simulink model "Final_prob"  (R2024b)
settings: Solver=VariableStepAuto  StartTime=0.0  StopTime=12  RelTol=1e-3
undefined symbols (not defined in the file or in its folder): A, B, C, D, sigbuilder_block
settings Model: Creator=shree  LastModifiedBy=shree

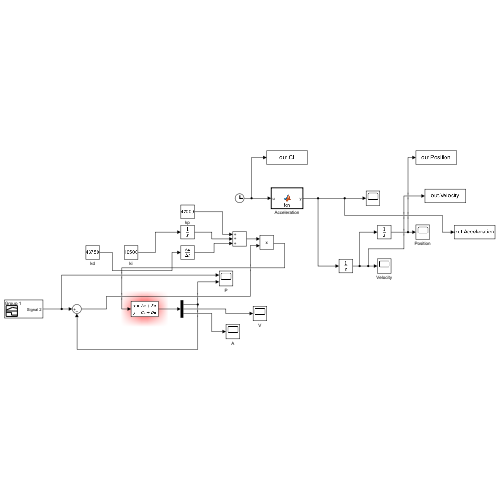
[thumbnail: Simulink's stored preview of the top-level diagram]
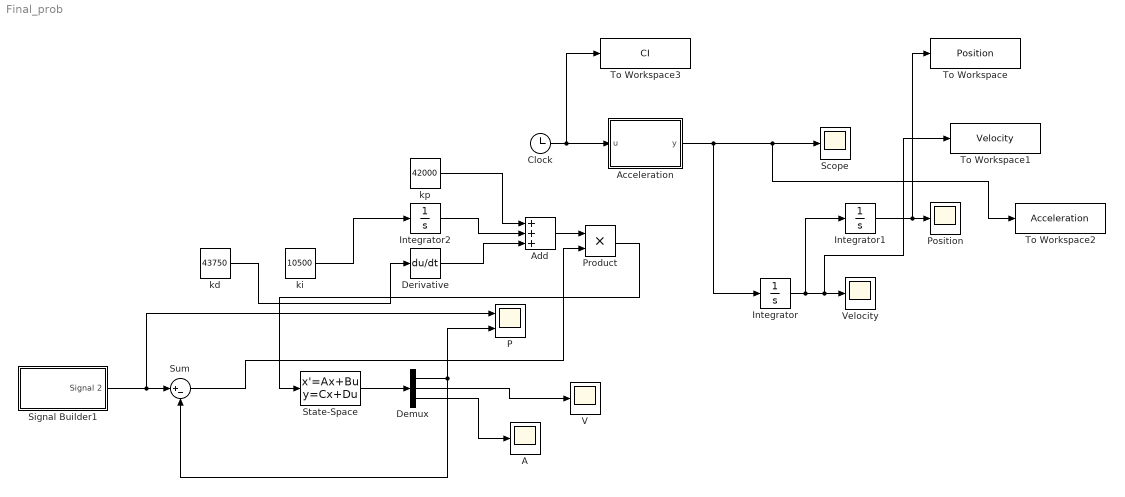
== system Final_prob ==
  A : Scope
  Acceleration : MATLAB Function  TreatAsAtomicUnit=on
  Add : Sum  Inputs=+++
  Clock : Clock
      settings: Decimation=12
  Demux : Demux  Outputs=3
  Derivative : Derivative
  Integrator : Integrator
  Integrator1 : Integrator
  Integrator2 : Integrator
  P : Scope  NumInputPorts=2
  Position : Scope
  Product : Product
  Scope : Scope
  Signal Builder1 : Subsystem  Tag=STV Subsys  LoadFcn=sigbuilder_block('load');  StartFcn=sigbuilder_block('start');  StopFcn=sigbuilder_block('stop');  ClipboardFcn=sigbuilder_block('clipboard');  mask(Sigbuilder block){tuvar=[0:10]}
      mask help: Simulink:masks:SigbuilderBlock_MD
      mask init:
      | if ~strcmp(get_param(bdroot(gcbh),'SimulationStatus'),'stopped') tuvar = sigbuilder_block('maskInit'); end
      settings: CopyFcn=sigbuilder_block('copy');  DeleteFcn=sigbuilder_block('delete');  ModelCloseFcn=sigbuilder_block('modelClose');  PreSaveFcn=sigbuilder_block('preSave');  PauseFcn=sigbuilder_block('pause');  ContinueFcn=sigbuilder_block('continue');  NameChangeFcn=sigbuilder_block('namechange');  OpenFcn=sigbuilder_block('open',[5.4 36 1141.2 516.6 ]);  CloseFcn=sigbuilder_block('close');
      mask Display: plot(0, 0, 100, 100,[2, 2, 32, 32, 2], [68, 8, 8, 68, 68],[32, 2], [38, 38], [32, 19, 2],[53, 60, 44], [32, 17, 17, 2],[16, 16, 31, 31]);txt = getActiveGroup(gcbh);text(2, 100, txt,'verticalAlignment', 'top');
  State-Space : StateSpace  A=A  B=B  C=C  D=D  InitialCondition=0
  Sum : Sum  Inputs=|+-
  To Workspace : ToWorkspace  VariableName=Position  SampleTime=-1
  To Workspace1 : ToWorkspace  VariableName=Velocity  SampleTime=-1
  To Workspace2 : ToWorkspace  VariableName=Acceleration  SampleTime=-1
  To Workspace3 : ToWorkspace  VariableName=CI  SampleTime=-1
  V : Scope
  Velocity : Scope
  kd : Constant  Value=43750
  ki : Constant  Value=10500
  kp : Constant  Value=42000
  wires:
  Acceleration/1(y) -> Integrator/1, To Workspace2/1, Scope/1
  Integrator/1 -> Integrator1/1, To Workspace1/1, Velocity/1
  Integrator1/1 -> To Workspace/1, Position/1
  Clock/1 -> To Workspace3/1, Acceleration/1(u)
  State-Space/1 -> Demux/1
  Demux/1 -> Sum/2, P/2
  Demux/2 -> V/1
  Signal Builder1/1(Signal 2) -> P/1, Sum/1
  Demux/3 -> A/1
  ki/1 -> Integrator2/1
  kd/1 -> Derivative/1
  Derivative/1 -> Add/3
  Integrator2/1 -> Add/2
  kp/1 -> Add/1
  Add/1 -> Product/1
  Sum/1 -> Product/2
  Product/1 -> State-Space/1

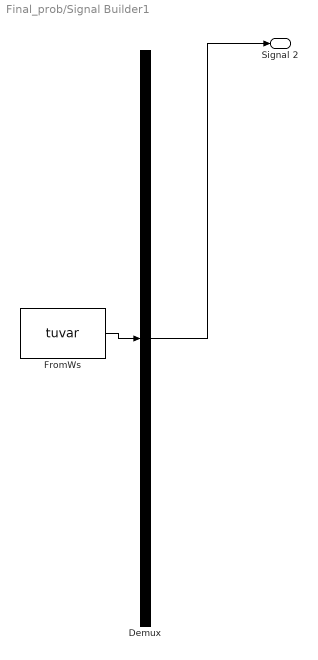
== system Final_prob/Signal Builder1 ==
  Demux : Demux  Tag=STV Demux  Outputs=1
      settings: DisplayOption=none
  FromWs : FromWorkspace  Tag=STV FromWs  VariableName=tuvar
      SigBuilderData=|
      | common.afterFinalStr = 'Extrapolate'
      | common.sampleTime = 0
      | dataSet.timeRange = [0 14]
      | dataSet.name = 'Group 1'
      | sbobj.Groups.Name = 'Group 1'
      | sbobj.Groups.Signals.Name = 'Signal 2'
      | sbobj.Groups.Signals.XData = [0 2 4 6 8 10 12 14]
      | sbobj.Groups.Signals.YData = [0 1 1 0 -1 -1 0 0]
      | sbobj.Groups.TimeRange = [0 14]
  Signal 2 : Outport  Tag=STV Outport
  wires:
  FromWs/1 -> Demux/1
  Demux/1 -> Signal 2/1

== matlab function Final_prob/Acceleration ==
  data: u input; y output
function y = fcn(u)
    x = zeros(size(u)); 
    if all(u >= 0 & u <= 4)
        x(u >= 0 & u <= 4) = 2.5 * u(u >= 0 & u <= 4) - 10;
    elseif all(u > 4 & u < 7)
        x(u > 4 & u < 7) = 0;
    elseif all(u >= 7 & u <= 12)
        x(u >= 7 & u <= 12) = 2 * u(u >= 7 & u <= 12) - 14;
    end
    y = x;
end
